simulink model "GFo_29bus"  (R2017b)
settings: Solver=ode1  StartTime=0.0  StopTime=4.5  FixedStep=Time_Step  RelTol=1e-3  EnableMultiTasking=on
PreLoadFcn:
  | Init_29bus;
InitFcn:
  | Init_29bus;
undefined symbols (not defined in the file): D1, D11, Delta, Time_Step, VSC01_Delta_P_Time_Step, VSC01_Delta_P_Value
libraries: powerlib x168, sps_avr x6, GFo_Lib x1
(part 1 of 5)
Description:
  | Copyright 2008-2017 The MathWorks, Inc.
settings Model: Creator=MathWorks  LastModifiedBy=Frederic_Colas
settings DataIOCC: SaveFormat=StructureWithTime  SignalLoggingSaveFormat=ModelDataLogs  SaveOutput=off  SignalLogging=off  DSMLogging=off  SaveTime=off
settings OptimizationCC: ExpressionDepthLimit=2147483647  LifeSpan=inf
settings DebuggingCC: UnderspecifiedInitializationDetection=Classic  MergeDetectMultiDrivingBlocksExec=none  SolverPrmCheckMsg=warning  FcnCallInpInsideContextMsg=warning  UnconnectedInputMsg=none  UnconnectedOutputMsg=none  UnconnectedLineMsg=none  StateNameClashWarn=warning  SFUnexpectedBacktrackingDiag=warning  SFNoUnconditionalDefaultTransitionDiag=warning  SFExecutionAtInitializationDiag=none
settings HardwareCC: ProdBitPerPointer=32  ProdBitPerSizeT=32  ProdBitPerPtrDiffT=32  ProdLargestAtomicFloat=None  ProdIntDivRoundTo=Undefined  ProdEndianess=Unspecified  ProdWordSize=32  ProdHWDeviceType=32-bit Generic
settings ModelReferenceCC: PropagateSignalLabelsOutOfModel=off
settings CodeAppCC: StateflowObjectComments=on
settings GRTTargetCC: TargetLangStandard=C89/C90 (ANSI)  GeneratePreprocessorConditionals=Disable all  CombineOutputUpdateFcns=off  GRTInterface=on
settings ConfigComp: CovMetricSettings=dw  CovHtmlReporting=on  CovSaveCumulativeToWorkspaceVar=on  CovSaveSingleToWorkspaceVar=on  CovExternalEMLEnable=off  CovSFcnEnable=off
settings SimscapeCC: SimscapeNormalizeSystem=off

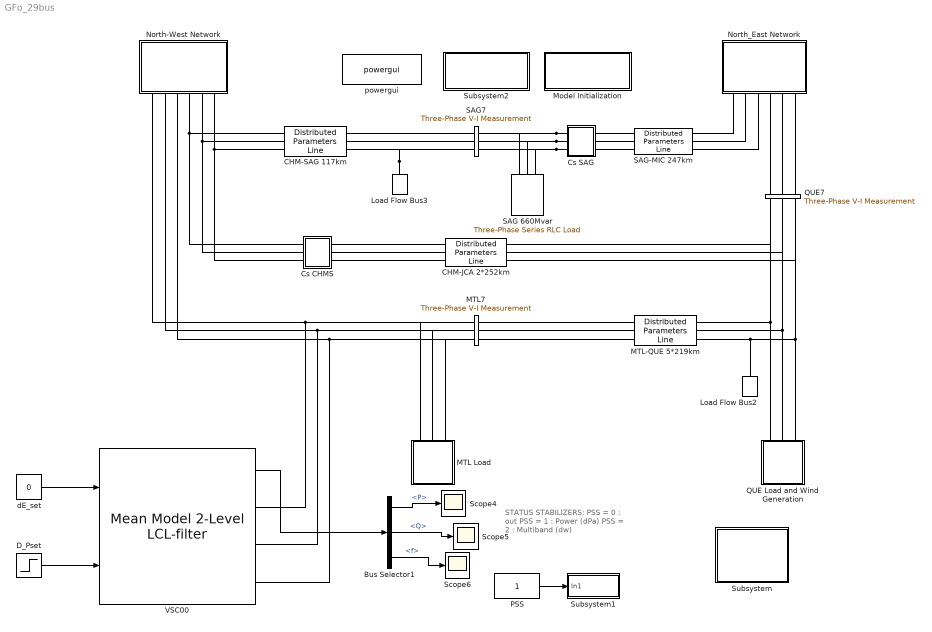
== system GFo_29bus ==
  note: STATUS STABILIZERS:
      | PSS = 0 :  out
      | PSS = 1 :  Power (dPa)
      | PSS = 2 :  Multiband (dw)
  Bus Selector1 : BusSelector  OutputSignals=control.P,control.Q,control.f
  CHM-JCA 2*252km : powerlib/Elements/Distributed Parameters Line  Phases=3  Frequency=60  Resistance="[0.01273  0.3864]/2"  Inductance="[0.9337e-3  4.1264e-3]/2"  Capacitance=[12.74e-9 7.751e-9]*2  Length=252  x1=[-0.00144 -1.85754414485872e-08 0 0;-0.0014 -1.70488676972424e-08 0 0;-0.00136 -1.55184171804064e-08 0 0;-0.00132 -1.39844379093287e-08 0 0;-0.00128 -1.2447278697667e-08 0 0;-0.00124 -1.09072890821703e-08 0 0;-0.0012 -9.36481924319672e-09 0 0;-0.00116 -7.82021992508601e-09 0 0;-0.00112 -6.27384235640306e-09 0 0;-0.00108 -4.72603817007156e-09 0 0;-0.00104 -3.17715932341582e-09 0 0;-0.001 -1.62755801812856e-09 0 0;-0.00096 -7.7586620183467e-11 0 0;-0.00092 1.47240242028999e-09 0 0;-0.00088 3.02205664915053e-09 172196.876340074 -778424.9668511;-0.00084 4.57102368839016e-09 183915.187892279 -775739.943274932;-0.0008 6.11895131626187e-09 195591.678716774 -772878.523125359;-0.00076 7.66548754737186e-09 207223.69368024 -769841.357064648;-0.00072 9.21028071271792e-09 218808.587762784 -766629.13571817;-0.00068 1.0752979539656e-08 230343.726659395 -763242.589517357;-0.00064 1.22932332317765e-08 241826.487378964 -759682.488533612;-0.0006 1.38306915486724e-08 253254.258840726 -755949.642303197;-0.00056 1.5365004885581e-08 264624.442467999 -752044.899643155;-0.00052 1.68958243528807e-08 275934.452779079 -747969.148458292;-0.00048 1.8422801855426e-08 287181.717975154 -743723.315539282;-0.00044 1.99455901717008e-08 298363.680525112 -739308.366351914;-0.0004 2.1463843032774e-08 309477.797747096 -734725.304817562;-0.00036 2.29772152010379e-08 320521.542386696 -729975.173084896;-0.00032 2.44853625487121e-08 331492.403191618 -725059.051292908;-0.00028 2.59879421360955e-08 342387.885482722 -719978.057325298;-0.00024 2.74846122895477e-08 353205.511721295 -714733.34655628;-0.0002 2.89750326791824e-08 363942.822072417 -709326.111587852;-0.00016 3.04588643962559e-08 374597.374964309 -703757.581978617;-0.00012 3.19357700302317e-08 385166.747643524 -698029.023964187;-8e-05 3.3405413745505e-08 395648.536725862 -692141.740169254;-4e-05 3.48674613577686e-08 406040.358742876 -686097.069311382]  x2=[-0.00144 -4.16824187889297e-09 0 0;-0.0014 -3.16521867758044e-09 0 0;-0.00136 -2.16147573283633e-09 0 0;-0.00132 -1.15724128715034e-09 0 0;-0.00128 -1.52743694775274e-10 0 0;-0.00124 8.51788630198777e-10 0 0;-0.0012 1.85612726578383e-09 0 0;-0.00116 2.86004383403521e-09 0 0;-0.00112 3.86331005298269e-09 0 0;-0.00108 4.8656977885399e-09 0 0;-0.00104 5.86697910637997e-09 0 0;-0.001 6.86692632376594e-09 0 0;-0.00096 7.86531206132372e-09 0 0;-0.00092 8.86190929474633e-09 0 0;-0.00088 9.85649140641716e-09 -50539.1882480982 -801013.244555649;-0.00084 1.08488322369409e-08 -38454.9386555758 -801684.296463899;-0.0008 1.18387061365704e-08 -26361.9447416245 -802173.052276564;-0.00076 1.2825888016517e-08 -14262.9563487746 -802479.400854788;-0.00072 1.38101534001344e-08 -2160.72468264951 -802603.272537544;-0.00068 1.47912784739624e-08 9941.99831363509 -802544.639157481;-0.00064 1.57690401386199e-08 22042.4605852394 -802303.514047325;-0.0006 1.67432160595363e-08 34137.9105913927 -801879.952036844;-0.00056 1.7713584717508e-08 46225.5979310702 -801274.049440389;-0.00052 1.86799254590705e-08 58302.7739684108 -800485.944034984;-0.00048 1.96420185466724e-08 70366.6924577328 -799515.815029002;-0.00044 2.05996452086424e-08 82414.6101680063 -798363.883021413;-0.0004 2.15525876889357e-08 94443.787506641 -797030.409951622;-0.00036 2.25006292966501e-08 106451.489142445 -795515.699039906;-0.00032 2.34435544552996e-08 118434.984627617 -793820.094718463;-0.00028 2.43811487518346e-08 130391.549018624 -791943.982553094;-0.00024 2.53131989853975e-08 142318.463495833 -789887.789155527;-0.0002 2.62394932158028e-08 154213.015981746 -787651.982086408;-0.00016 2.71598208117306e-08 166072.5017577 -785237.069748983;-0.00012 2.80739724986222e-08 177894.224078904 -782643.601273494;-8e-05 2.89817404062672e-08 189675.494787646 -779872.166392307;-4e-05 2.98829181160717e-08 201413.634924565 -776923.395305812]  x3=[-0.00144 6.24964800002417e-11 0 0;-0.0014 6.65040601264245e-11 0 0;-0.00136 7.0496517802841e-11 0 0;-0.00132 7.44729451790454e-11 0 0;-0.00128 7.84324380497433e-11 0 0;-0.00124 8.23740960604013e-11 0 0;-0.0012 8.62970229119791e-11 0 0;-0.00116 9.02003265647405e-11 0 0;-0.00112 9.40831194410956e-11 0 0;-0.00108 9.7944518627428e-11 0 0;-0.00104 1.01783646074862e-10 0 0;-0.001 1.05599628798924e-10 0 0;-0.00096 1.09391599078049e-10 0 0;-0.00092 1.13158694650896e-10 0 0;-0.00088 1.16900058912419e-10 -378.521018352371 -850.366045683333;-0.00084 1.20614841108649e-10 -365.655684342529 -855.977425052353;-0.0008 1.24302196530148e-10 -352.707203383348 -861.394162536551;-0.00076 1.27961286704093e-10 -339.678519847734 -866.615026416536;-0.00072 1.31591279584933e-10 -326.57259634597 -871.638829512882;-0.00068 1.3519134974359e-10 -313.392413052039 -876.464429456091;-0.00064 1.38760678555156e-10 -300.140967025961 -881.090728946349;-0.0006 1.42298454385039e-10 -286.821271532287 -885.516676003047;-0.00056 1.45803872773525e-10 -273.436355354908 -889.741264203993;-0.00052 1.49276136618702e-10 -259.989262108336 -893.763532914261;-0.00048 1.52714456357713e-10 -246.483049545612 -897.582567504632;-0.00044 1.56118050146303e-10 -232.920788863001 -901.197499559575;-0.0004 1.59486144036594e-10 -219.305564001625 -904.607507074715;-0.00036 1.6281797215308e-10 -205.640470946207 -907.811814643748;-0.00032 1.66112776866782e-10 -191.928617021063 -910.809693634768;-0.00028 1.6936980896752e-10 -178.17312018353 -913.600462355943;-0.00024 1.72588327834281e-10 -164.377108314967 -916.183486210533;-0.0002 1.75767601603632e-10 -150.543718509501 -918.558177841189;-0.00016 1.78906907336133e-10 -136.67609636068 -920.723997263512;-0.00012 1.82005531180733e-10 -122.777395246191 -922.680451988843;-8e-05 1.85062768537091e-10 -108.85077561081 -924.427097136249;-4e-05 1.88077924215798e-10 -94.8994042477446 -925.963535533686]  x4=[-0.00144 -2.38829442616442e-10 0 0;-0.0014 -2.36838630214904e-10 0 0;-0.00136 -2.34793962751264e-10 0 0;-0.00132 -2.32695905165271e-10 0 0;-0.00128 -2.30544934537127e-10 0 0;-0.00124 -2.28341539979005e-10 0 0;-0.0012 -2.26086222523825e-10 0 0;-0.00116 -2.23779495011327e-10 0 0;-0.00112 -2.21421881971456e-10 0 0;-0.00108 -2.19013919505086e-10 0 0;-0.00104 -2.16556155162116e-10 0 0;-0.001 -2.14049147816963e-10 0 0;-0.00096 -2.11493467541477e-10 0 0;-0.00092 -2.08889695475315e-10 0 0;-0.00088 -2.06238423693789e-10 -648.242255193202 -10861.6585886729;-0.00084 -2.0354025507324e-10 -484.384788092552 -10870.1989782703;-0.0008 -2.00795803153944e-10 -320.417176068246 -10876.2675783607;-0.00076 -1.980056920006e-10 -156.376703941262 -10879.8630089967;-0.00072 -1.95170556060423e-10 7.69932689966229 -10880.9844526083;-0.00068 -1.92291040018877e-10 171.773606980046 -10879.6316541891;-0.00064 -1.89367798653078e-10 335.808827223516 -10875.8049213537;-0.0006 -1.86401496682904e-10 499.767687435566 -10869.5051242681;-0.00056 -1.83392808619843e-10 663.612904785307 -10860.7336954518;-0.00052 -1.80342418613613e-10 827.307222283253 -10849.4926294522;-0.00048 -1.77251020296597e-10 990.813417253246 -10835.7844823907;-0.00044 -1.74119316626114e-10 1154.09430979657 -10819.6123713818;-0.0004 -1.70948019724571e-10 1317.11277124632 -10800.9799738239;-0.00036 -1.67737850717535e-10 1479.8317326102 -10779.8915265637;-0.00032 -1.64489539569756e-10 1642.2141929996 -10756.3518249321;-0.00028 -1.61203824919176e-10 1804.22322804337 -10730.3662216544;-0.00024 -1.57881453908972e-10 1965.82199828404 -10701.9406256326;-0.0002 -1.54523182017661e-10 2126.97375755482 -10671.0815006022;-0.00016 -1.5112977288731e-10 2287.64186133538 -10637.795863662;-0.00012 -1.47701998149892e-10 2447.78977508446 -10602.0912836789;-8e-05 -1.44240637251823e-10 2607.38108254751 -10563.9758795664;-4e-05 -1.40746477276721e-10 2766.3794940375 -10523.4583184387]  x5=0.00142516474882927  V1=ones(3,3)  V2=ones(3,3)  I1=ones(3,3)  I2=ones(3,3)  nHarmo=1  Measurements=None
      settings: AttributesFormatString=\n  SourceProductName=Simscape Power Systems
  CHM-SAG 117km : powerlib/Elements/Distributed Parameters Line  Phases=3  Frequency=60  Resistance="[0.01273  0.3864]"  Inductance="[0.9337e-3  4.1264e-3]"  Capacitance=[12.74e-9 7.751e-9]  Length=117  x1=[-0.00068 1.03484332071882e-08 0 0;-0.00064 1.18635422964804e-08 0 0;-0.0006 1.33759537185611e-08 0 0;-0.00056 1.48853235641156e-08 0 0;-0.00052 1.63913086154571e-08 0 0;-0.00048 1.78935664245721e-08 0 0;-0.00044 1.93917553909897e-08 223467.945952777 -779436.69611525;-0.0004 2.08855348394588e-08 235195.677690823 -775978.427940146;-0.00036 2.23745650974146e-08 246869.927960004 -772343.708962281;-0.00032 2.38585075722172e-08 258488.042136482 -768533.365685406;-0.00028 2.53370248281449e-08 270047.378361284 -764548.264548724;-0.00024 2.68097806631239e-08 281545.308141037 -760389.311729867;-0.0002 2.82764401851778e-08 292979.216945661 -756057.452938841;-0.00016 2.97366698885793e-08 304346.504802897 -751553.673202978;-0.00012 3.11901377296862e-08 315644.586889514 -746878.996642952;-8e-05 3.26365132024456e-08 326870.894119075 -742034.486239899;-4e-05 3.40754674135481e-08 338022.873726127 -737021.243593708]  x2=[-0.00068 7.57652475797684e-09 0 0;-0.00064 8.6127901811104e-09 0 0;-0.0006 9.64709713003032e-09 0 0;-0.00056 1.06792104122559e-08 0 0;-0.00052 1.17088953341273e-08 0 0;-0.00048 1.2735917754173e-08 0 0;-0.00044 1.37600441363512e-08 265658.843850609 -751135.268348524;-0.0004 1.47810416031544e-08 276955.015824463 -747044.008737732;-0.00036 1.57986779885633e-08 288188.210616077 -742782.877761587;-0.00032 1.68127218908396e-08 299355.873893826 -738352.844364525;-0.00028 1.78229427251446e-08 310455.466227387 -733754.915897938;-0.00024 1.88291107759725e-08 321484.463665181 -728990.137891109;-0.0002 1.98309972493853e-08 332440.358308303 -724059.593813467;-0.00016 2.08283743250387e-08 343320.658880788 -718964.404828216;-0.00012 2.1821015207987e-08 354122.891296115 -713705.729537391;-8e-05 2.28086941802533e-08 364844.599219787 -708284.763718406;-4e-05 2.37911866521568e-08 375483.344627883 -702702.740052139]  x3=[-0.00068 1.54291039105485e-10 0 0;-0.00064 1.55495560223311e-10 0 0;-0.0006 1.56664722991678e-10 0 0;-0.00056 1.57798261553056e-10 0 0;-0.00052 1.58895918150551e-10 0 0;-0.00048 1.59957443186519e-10 0 0;-0.00044 1.6098259527932e-10 1327.17874386151 -3929.54387650929;-0.0004 1.6197114131821e-10 1386.28134396302 -3909.08471567241;-0.00036 1.62922856516344e-10 1445.0687156417 -3887.73666268169;-0.00032 1.63837524461892e-10 1503.52749115618 -3865.50457190029;-0.00028 1.64714937167253e-10 1561.64437748503 -3842.39349871393;-0.00024 1.65554895116343e-10 1619.4061593495 -3818.40869838136;-0.0002 1.66357207309968e-10 1676.79970221849 -3793.55562483933;-0.00016 1.67121691309254e-10 1733.81195529531 -3767.83992946244;-0.00012 1.67848173277132e-10 1790.42995448525 -3741.26745977806;-8e-05 1.68536488017869e-10 1846.64082534354 -3713.84425813664;-4e-05 1.69186479014627e-10 1902.43178600291 -3685.57656033774]  x4=[-0.00068 -1.5758176037485e-10 0 0;-0.00064 -1.55417777405434e-10 0 0;-0.0006 -1.53218453773701e-10 0 0;-0.00056 -1.50984289586881e-10 0 0;-0.00052 -1.48715792874641e-10 0 0;-0.00048 -1.46413479473572e-10 0 0;-0.00044 -1.44077872909887e-10 42.4498796181136 -1838.17704499413;-0.0004 -1.41709504280376e-10 70.1631282495175 -1837.32799490434;-0.00036 -1.39308912131643e-10 97.8604223906187 -1836.06115227294;-0.00032 -1.3687664233764e-10 125.535463915581 -1834.37680516904;-0.00028 -1.34413247975544e-10 153.18195975862 -1832.27533659864;-0.00024 -1.31919289199988e-10 180.793623344995 -1829.75722441756;-0.0002 -1.29395333115692e-10 208.364176020519 -1826.8230412228;-0.00016 -1.26841953648503e-10 235.887348479272 -1823.47345422233;-0.00012 -1.24259731414893e-10 263.356882189187 -1819.70922508332;-8e-05 -1.21649253589929e-10 290.766530815185 -1815.53120975904;-4e-05 -1.19011113773758e-10 318.11006163954 -1810.94035829413]  x5=0.000661683633385019  V1=ones(3,3)  V2=ones(3,3)  I1=ones(3,3)  I2=ones(3,3)  nHarmo=1  Measurements=None
      settings: AttributesFormatString=\n  SourceProductName=Simscape Power Systems
  Cs CHMS : Subsystem  mask{Xc=33/2}
      mask prompts: Xc "Condensator Reactance at  60Hz  (ohm):"
      mask help: Series Compensation
      mask init:
      | Cs=1/Xc/(2*pi*60);
      mask Display: disp('Cs')
  Cs SAG : Subsystem  mask{Xc=22}
      mask prompts: Xc "Condensator Reactance at  60Hz  (ohm):"
      mask help: Series Compensation
      mask init:
      | Cs=1/Xc/(2*pi*60);
      mask Display: disp('Cs')
  D_Pset : Step  Time=VSC01_Delta_P_Time_Step  After=VSC01_Delta_P_Value  SampleTime=0
  Load Flow Bus2 : powerlib/Measurements/Load Flow Bus  LConnTagsString=a  Phases=single  Connectors=on one side  ID=QUE7  Vbase=735e3  Vref=1  Vangle=0  VLF=1.092  VLFb=1  VLFc=1  angleLF=-14.6  angleLFb=0  angleLFc=0
      settings: AttributesFormatString=%<ID>\n%<Vbase>V\n%<VLF>pu\n%<angleLF>deg.  SourceProductName=Simscape Power Systems
  Load Flow Bus3 : powerlib/Measurements/Load Flow Bus  LConnTagsString=a  Phases=single  Connectors=on one side  ID=SAG7  Vbase=735e3  Vref=1  Vangle=0  VLF=1.084  VLFb=1  VLFc=1  angleLF=-1.02  angleLFb=0  angleLFc=0
      settings: AttributesFormatString=%<ID>\n%<Vbase>V\n%<VLF>pu\n%<angleLF>deg.  SourceProductName=Simscape Power Systems
  MTL Load : Subsystem
  MTL-QUE 5*219km : powerlib/Elements/Distributed Parameters Line  Phases=3  Frequency=60  Resistance="[0.01273  0.3864]/5"  Inductance="[0.9337e-3  4.1264e-3]/5"  Capacitance=[12.74e-9 7.751e-9]*5  Length=219  x1=[-0.00124 -5.4468796144153e-08 -263340.269226421 -757862.009549339;-0.0012 -4.83459032566071e-08 -251882.489501348 -761746.813211586;-0.00116 -4.2212016927578e-08 -240367.433870303 -765458.402217534;-0.00112 -3.60685319499204e-08 -228797.720757637 -768995.932583849;-0.00108 -2.99168452991393e-08 -217175.981016339 -772358.599906634;-0.00104 -2.3758355815729e-08 -205504.857329803 -775545.639544336;-0.001 -1.75944638870895e-08 -193787.003610908 -778556.326791627;-0.00096 -1.14265711290903e-08 -182025.084398541 -781389.97704419;-0.00092 -5.25608006735493e-09 -170221.774251699 -784045.945954392;-0.00088 9.15606181661316e-10 -158379.757141321 -786523.629577809;-0.00084 7.08708422972765e-09 -146501.725839979 -788822.464510551;-0.0008 1.32569507359566e-08 -134590.381309558 -790941.928017378;-0.00076 1.94238027259112e-08 -122648.432087085 -792881.538150567;-0.00072 2.55862379106297e-08 -110678.593668831 -794640.8538595;-0.00068 3.17428550054937e-08 -98683.5878928278 -796219.475090956;-0.00064 3.78922540488681e-08 -86666.1423199488 -797617.04288008;-0.0006 4.40330367204407e-08 -74628.9896136833 -798833.23943201;-0.00056 5.01638066591878e-08 -62574.8669187526 -799867.788194138;-0.00052 5.62831697808949e-08 -50506.5152387072 -800720.453918996;-0.00048 6.23897345951591e-08 -38426.6788126462 -801391.042717752;-0.00044 6.84821125218026e-08 -26338.1044912007 -801879.402104296;-0.0004 7.45589182066232e-08 -14243.5411119241 -802185.421029915;-0.00036 8.06187698364124e-08 -2145.73887422974 -802309.029908544;-0.00032 8.66602894531674e-08 9952.55128598059 -802250.200632591;-0.00028 9.26821032674272e-08 22048.5783218556 -802008.946579325;-0.00024 9.86828419706605e-08 34139.5917011591 -801585.322607837;-0.0002 1.04661141046634e-07 46222.8420317171 -800979.425046565;-0.00016 1.10615641081693e-07 58295.5816866058 -800191.391671391;-0.00012 1.16544988073879e-07 70355.0654289387 -799221.401674307;-8e-05 1.22447833740818e-07 82398.5510361093 -798069.675622674;-4e-05 1.28322835826309e-07 94423.2999233492 -796736.475409064]  x2=[-0.00124 9.0375128968403e-10 -158451.694559255 -786809.273834629;-0.0012 1.9084795416908e-09 -146569.352833624 -789109.165478305;-0.00116 2.91277382190782e-09 -134653.682501119 -791229.620502738;-0.00112 3.91640576247643e-09 -122707.393082416 -793170.156734742;-0.00108 4.91914714614829e-09 -110733.201060711 -794930.332913113;-0.00104 5.92076995818004e-09 -98733.8292640061 -796509.748788967;-0.001 6.92104643818184e-09 -86712.0062459713 -797908.045216754;-0.00096 7.91974913190816e-09 -74670.4656654886 -799124.904235924;-0.00092 8.91665094297889e-09 -62611.9456650443 -800160.049143231;-0.00088 9.91152518451912e-09 -50539.1882480981 -801013.244555649;-0.00084 1.09041456307057e-08 -38454.9386555758 -801684.296463899;-0.0008 1.18942865682093e-08 -26361.9447416244 -802173.052276565;-0.00076 1.28817228475192e-08 -14262.9563487745 -802479.400854788;-0.00072 1.38662299341408e-08 -2160.72468264948 -802603.272537544;-0.00068 1.48475839596526e-08 9941.99831363515 -802544.639157482;-0.00064 1.58255617726122e-08 22042.4605852394 -802303.514047325;-0.0006 1.67999409892985e-08 34137.9105913927 -801879.952036844;-0.00056 1.77705000442803e-08 46225.5979310702 -801274.049440389;-0.00052 1.87370182407984e-08 58302.7739684108 -800485.944034984;-0.00048 1.96992758009496e-08 70366.6924577328 -799515.815029002;-0.00044 2.0657053915663e-08 82414.6101680063 -798363.883021413;-0.0004 2.16101347944549e-08 94443.787506641 -797030.409951622;-0.00036 2.25583017149523e-08 106451.489142445 -795515.699039906;-0.00032 2.35013390721743e-08 118434.984627617 -793820.094718463;-0.00028 2.44390324275582e-08 130391.549018624 -791943.982553094;-0.00024 2.53711685577213e-08 142318.463495833 -789887.789155527;-0.0002 2.6297535502946e-08 154213.015981746 -787651.982086408;-0.00016 2.72179226153777e-08 166072.5017577 -785237.069748984;-0.00012 2.81321206069239e-08 177894.224078904 -782643.601273495;-8e-05 2.90399215968453e-08 189675.494787646 -779872.166392307;-4e-05 2.99411191590251e-08 201413.634924565 -776923.395305813]  x3=[-0.00124 3.81189466927696e-09 -8469.52016261608 -20114.2598393833;-0.0012 3.84351344492956e-09 -8165.25294654191 -20239.6869599555;-0.00116 3.87425823876983e-09 -7859.12902236185 -20360.5117502527;-0.00112 3.90412205969678e-09 -7551.21800001634 -20476.7067357594;-0.00108 3.93309811693508e-09 -7241.58989581657 -20588.245494738;-0.00104 3.96117982157917e-09 -6930.31511652329 -20695.1026642366;-0.001 3.9883607880916e-09 -6617.46444333701 -20797.2539458563;-0.00096 4.01463483575498e-09 -6303.10901580289 -20894.6761112766;-0.00092 4.03999599007744e-09 -5987.32031563429 -20987.3470075372;-0.00088 4.0644384841512e-09 -5670.17015045835 -21075.2455620755;-0.00084 4.08795675996389e-09 -5351.73063748767 -21158.3517875181;-0.0008 4.1105454696624e-09 -5032.07418712138 -21236.6467862261;-0.00076 4.13219947676895e-09 -4711.2734864797 -21310.112754592;-0.00072 4.15291385734904e-09 -4389.40148287549 -21378.732987088;-0.00068 4.17268390113118e-09 -4066.53136722666 -21442.4918800651;-0.00064 4.1915051125779e-09 -3742.73655741319 -21501.3749353009;-0.0006 4.20937321190802e-09 -3418.09068158255 -21555.3687632963;-0.00056 4.22628413606983e-09 -3092.66756140728 -21604.4610863206;-0.00052 4.24223403966503e-09 -2766.54119529857 -21648.6407412027;-0.00048 4.25721929582308e-09 -2439.78574157969 -21687.8976818703;-0.00044 4.27123649702595e-09 -2112.47550162299 -21722.2229816334;-0.0004 4.28428245588297e-09 -1784.68490295443 -21751.608835215;-0.00036 4.2963542058556e-09 -1456.48848232941 -21776.0485605253;-0.00032 4.307449001932e-09 -1127.96086878373 -21795.5366001817;-0.00028 4.31756432125122e-09 -799.176766663608 -21810.0685227718;-0.00024 4.32669786367688e-09 -470.210938638553 -21819.6410238619;-0.0002 4.33484755232019e-09 -141.138188700978 -21824.2519267477;-0.00016 4.34201153401224e-09 187.966654843584 -21823.9001829498;-0.00012 4.34818817972536e-09 517.02875639179 -21818.5858724515;-8e-05 4.35337608494359e-09 845.973290059458 -21808.3102036813;-4e-05 4.35757406998203e-09 1174.72545669633 -21793.0755132376]  x4=[-0.00124 -4.87811680086981e-09 -3328.85135662787 -7082.90675391454;-0.0012 -4.86617754969349e-09 -3221.66969661535 -7132.29763529397;-0.00116 -4.85313177170651e-09 -3113.75545669631 -7180.06669369745;-0.00112 -4.83898243340626e-09 -3005.13317563831 -7226.20306685304;-0.00108 -4.82373275223026e-09 -2895.82755321133 -7270.69626374736;-0.00104 -4.80738619582451e-09 -2785.8634445713 -7313.5361670111;-0.001 -4.78994648125495e-09 -2675.26585460824 -7354.71303521972;-0.00096 -4.7714175741623e-09 -2564.05993226035 -7394.21750510848;-0.00092 -4.75180368786024e-09 -2452.27096479538 -7432.04059370159;-0.00088 -4.73110928237737e-09 -2339.9243720605 -7468.17370035488;-0.00084 -4.70933906344303e-09 -2227.04570070206 -7502.6086087115;-0.0008 -4.68649798141728e-09 -2113.6606183565 -7535.33748857023;-0.00076 -4.66259123016519e-09 -1999.79490781376 -7566.35289766605;-0.00072 -4.63762424587583e-09 -1885.47446115448 -7595.64778336239;-0.00068 -4.61160270582614e-09 -1770.72527386238 -7623.21548425487;-0.00064 -4.5845325270899e-09 -1655.57343891308 -7649.04973168604;-0.0006 -4.55641986519233e-09 -1540.04514084083 -7673.14465117082;-0.00056 -4.52727111271031e-09 -1424.16664978434 -7695.4947637323;-0.00052 -4.49709289781877e-09 -1307.96431551318 -7716.09498714764;-0.00048 -4.46589208278356e-09 -1191.46456143607 -7734.94063710366;-0.00044 -4.43367576240093e-09 -1074.69387859244 -7752.02742826209;-0.0004 -4.40045126238432e-09 -957.678819628593 -7767.35147523398;-0.00036 -4.36622613769852e-09 -840.445992759828 -7780.90929346318;-0.00032 -4.33100817084174e-09 -723.022055720008 -7792.69780001875;-0.00028 -4.29480537007593e-09 -605.433709699793 -7802.71431429596;-0.00024 -4.25762596760579e-09 -487.707693275031 -7810.95655862585;-0.0002 -4.21947841770682e-09 -369.87077632663 -7817.42265879312;-0.00016 -4.1803713948029e-09 -251.949753953322 -7822.11114446236;-0.00012 -4.14031379149379e-09 -133.971440378687 -7825.02094951237;-8e-05 -4.09931471653303e-09 -15.96266285383 -7826.15141227857;-4e-05 -4.05738349275672e-09 102.049744442903 -7825.50227570347]  x5=0.00123853603172068  V1=ones(3,3)  V2=ones(3,3)  I1=ones(3,3)  I2=ones(3,3)  nHarmo=1  Measurements=None
      settings: AttributesFormatString=\n  SourceProductName=Simscape Power Systems
  MTL7 : powerlib/Measurements/Three-Phase V-I Measurement  VoltageMeasurement=phase-to-ground  SetLabelV=on  LabelV=Vabc_MTL7  Vpu=on  VpuLL=off  CurrentMeasurement=no  SetLabelI=off  LabelI=A1  Ipu=off  Pbase=100e6  Vbase=735e3  OutputType=Magnitude  PhasorSimulation=off  PSBequivalent=0
  Model Initialization : Subsystem  mask(Model Functions){InitFcnX=Init_29bus;, prel=on, posl=off, inif=on, strf=off}
      mask prompts: InitFcnX "Initialisation"; prel "Preload Function"; posl "PostLoad Function"; inif "InitFcn"; strf "StartFcn"
      mask init:
      | currentBlock = gcb;
      | root = bdroot(currentBlock);
      | 
      | if ~strcmp(get_param(root,'BlockDiagramType'),'library')
      |     if prel==1
      |         set_param(root, 'PreLoadFcn', InitFcnX);
      |     else
      |         set_param(root, 'PreLoadFcn', '');
      |     end
      |     if inif==1
      |         set_param(root, 'InitFcn', InitFcnX);
      |     else
      |         set_param(root, 'InitFcn', '');
      |     end
      |     if strf==1
      |         set_param(root, 'StartFcn', InitFcnX);
      |     else
      |         set_param(root, 'StartFcn', '');
      |     end
      |     if posl==1
      |         set_param(root, 'PostLoadFcn', InitFcnX);
      |     else
      |         set_param(root, 'PostLoadFcn', '');
      |     end
      | end
      | 
      | pos = get_param(currentBlock, 'Position');
      | width = pos(3) - pos(1); height = pos(4) - pos(2);
      | txt = [ upper(root) '\n' '- InitFcn. . . . . '  get_param(root, 'InitFcn') ];
      settings: CopyFcn=set_param(gcb,'LinkStatus','none')
      mask Display:
      | %text(5, height*0.5, txt, 'horizontalAlignment', 'left', 'verticalAlignment', 'middle') ;
      | color('blue'),disp('Initialization Function\nParameters')
  North-West Network : Subsystem
  North_East Network : Subsystem
  PSS : Constant
  QUE Load and Wind Generation : Subsystem
  QUE7 : powerlib/Measurements/Three-Phase V-I Measurement  VoltageMeasurement=no  SetLabelV=on  LabelV=Vabc_QUE7  Vpu=on  VpuLL=off  CurrentMeasurement=no  SetLabelI=off  LabelI=A1  Ipu=off  Pbase=100e6  Vbase=735e3  OutputType=Magnitude  PhasorSimulation=off  PSBequivalent=0
  SAG 660Mvar : powerlib/Elements/Three-Phase Series RLC Load  LConnTagsString=A|B|C  Configuration=Y (grounded)  NominalVoltage=735e3  Vabc=[1e3 1e3 1e3]  Vabcp=[1e3 1e3 1e3]  NominalFrequency=60  UnbalancedPower=off  ActivePower=2200000  InductivePower=660e6  CapacitivePower=0  Pabc=[10e3 9e3 11e3]  QLabc=[100 90 110]  QCabc=[100 90 110]  Pabcp=[10e3 9e3 11e3]  QLabcp=[100 90 110]  QCabcp=[100 90 110]  Measurements=None  LoadType=constant Z
  SAG-MIC 247km : powerlib/Elements/Distributed Parameters Line  Phases=3  Frequency=60  Resistance="[0.01273  0.3864]/1"  Inductance="[0.9337e-3  4.1264e-3]/1"  Capacitance=[12.74e-9 7.751e-9]*1  Length=247  x1=[-0.0014 -1.08735468814976e-08 -43484.2882453679 -787188.223839926;-0.00136 -9.81375428176395e-09 -31609.3049024198 -787754.475242769;-0.00132 -8.75173011893683e-09 -19727.1338761239 -788141.598071246;-0.00128 -7.68771588815238e-09 -7840.47706970408 -788349.504296966;-0.00124 -6.62195353707101e-09 4047.96259358793 -788378.146643845;-0.0012 -5.55468541086059e-09 15935.4817850944 -788227.518598861;-0.00116 -4.48615419708932e-09 27819.3773854646 -787897.654413532;-0.00112 -3.41660287054057e-09 39696.9470993214 -787388.62909613;-0.00108 -2.3462746379626e-09 51565.4900697397 -786700.558394621;-0.00104 -1.27541288276536e-09 63422.307492398 -785833.59877035;-0.001 -2.04261109677269e-10 75264.7032292633 -784787.947362459;-0.00096 8.66937110625693e-10 87089.9844216694 -783563.841943061;-0.00092 1.93793819690584e-09 98895.46210265 -782161.560863172;-0.00088 3.00849861275208e-09 110678.451808387 -780581.422989417;-0.00084 4.07837492195797e-09 122436.274188632 -778823.787631521;-0.0008 5.14732384387701e-09 134166.255615973 -776889.054460608;-0.00076 6.21510230874259e-09 145865.728793787 -774777.663418317;-0.00072 7.28146751293991e-09 157532.033362766 -772490.094616762;-0.00068 8.34617697421749e-09 169162.516505857 -770026.868229362;-0.00064 9.40898858682551e-09 180754.533551489 -767388.544372556;-0.0006 1.04696606765685e-08 192305.448574953 -764575.722978437;-0.00056 1.15279520557602e-08 203812.634997782 -761589.043658332;-0.00052 1.25836220780673e-08 215273.476185018 -758429.185557364;-0.00048 1.36364306932303e-08 226685.366040209 -755096.867200015;-0.00044 1.46861385016492e-08 238045.709598014 -751592.846326742;-0.0004 1.57325068088207e-08 249351.923614275 -747917.919721676;-0.00036 1.67752976796153e-08 260601.437153426 -744072.923031434;-0.00032 1.78142739923815e-08 271791.692173099 -740058.730575107;-0.00028 1.88491994928657e-08 282920.144105803 -735876.255145441;-0.00024 1.98798388479337e-08 293984.262437537 -731526.447801282;-0.0002 2.09059576990841e-08 304981.531283206 -727010.297651308;-0.00016 2.1927322715739e-08 315909.449958709 -722328.831629118;-0.00012 2.29437016483016e-08 326765.533549578 -717483.114259714;-8e-05 2.39548633809674e-08 337547.313476025 -712474.247417439;-4e-05 2.49605779842783e-08 348252.338054271 -707303.370075417]  x2=[-0.0014 -1.04301270405993e-09 59840.985994314 -786906.914710697;-0.00136 -6.98506067436651e-10 71699.9647213889 -785915.133906567;-0.00132 -3.53840596557298e-10 83542.6394948002 -784744.642778429;-0.00128 -9.09466537767774e-12 95366.3173924316 -783395.707485873;-0.00124 3.35653333850417e-10 107168.309811892 -781868.634765151;-0.0012 6.80325008404946e-10 118945.933081881 -780163.771859432;-0.00116 1.02484198291944e-09 130696.509072434 -778281.506439838;-0.00112 1.36912591720487e-09 142417.365803902 -776222.266517293;-0.00108 1.71309852406357e-09 154105.838054541 -773986.520345198;-0.00104 2.05668158709104e-09 165759.267966559 -771574.776312952;-0.001 2.39979697846166e-09 177375.005650489 -768987.58283035;-0.00096 2.74236667669435e-09 188950.40978775 -766225.528202878;-0.00092 3.08431278439393e-09 200482.848231265 -763289.240497941;-0.00088 3.42555754596431e-09 211969.698603982 -760179.387402041;-0.00084 3.76602336528949e-09 223408.348895185 -756896.676068953;-0.0008 4.10563282337821e-09 234796.198054442 -753441.852958926;-0.00076 4.44430869596836e-09 246130.656583056 -749815.703668943;-0.00072 4.78197397108713e-09 257409.147122905 -746019.05275408;-0.00068 5.11855186656286e-09 268629.105042499 -742052.763540015;-0.00064 5.45396584748465e-09 279787.979020166 -737917.737926711;-0.0006 5.78813964360572e-09 290883.231624192 -733614.916183335;-0.00056 6.12099726668663e-09 301912.339889817 -729145.276734444;-0.00052 6.45246302777432e-09 312872.795892932 -724509.835937505;-0.00048 6.78246155441317e-09 323762.107320361 -719709.64785178;-0.00044 7.110917807784e-09 334577.798036591 -714745.803998646;-0.0004 7.43775709976728e-09 345317.408646824 -709619.433113387;-0.00036 7.76290510992657e-09 355978.49705622 -704331.700888536;-0.00032 8.08628790240829e-09 366558.639025214 -698883.809708801;-0.00028 8.40783194275419e-09 377055.428720761 -693276.998377655;-0.00024 8.72746411462236e-09 387466.479263404 -687512.541835644;-0.0002 9.04511173641331e-09 397789.423270032 -681591.750870476;-0.00016 9.36070257779712e-09 408021.913392197 -675515.971818956;-0.00012 9.674164876138e-09 418161.622849888 -669286.586260847;-8e-05 9.98542735281249e-09 428206.245960616 -662905.010704703;-4e-05 1.02944192294176e-08 438153.498663705 -656372.696265775]  x3=[-0.0014 8.14598994752012e-11 -581.71165728291 -4056.93337045252;-0.00136 8.26501374952971e-11 -520.470981275651 -4065.24415192315;-0.00132 8.3821581586871e-11 -459.1119546556 -4072.63053193081;-0.00128 8.49739653736386e-11 -397.648529936272 -4079.09083087638;-0.00124 8.61070268134644e-11 -336.094683370413 -4084.62357974358;-0.0012 8.72205082579483e-11 -274.464411771912 -4089.22752043305;-0.00116 8.83141565110119e-11 -212.771729333055 -4092.90160604837;-0.00112 8.93877228864738e-11 -151.030664437812 -4095.64500113415;-0.00108 9.04409632645982e-11 -89.2552564719097 -4097.45708186601;-0.00104 9.14736381476058e-11 -27.4595526303898 -4098.33743619242;-0.001 9.24855127141338e-11 34.3423952765968 -4098.2858639284;-0.00096 9.34763568726316e-11 96.1365340190545 -4097.30237680103;-0.00092 9.44459453136824e-11 157.908812142722 -4095.38719844681;-0.00088 9.5394057561236e-11 219.645183164256 -4092.54076436077;-0.00084 9.63204780227435e-11 281.331608765277 -4088.76372179749;-0.0008 9.7224996038181e-11 342.954061984566 -4084.05692962387;-0.00076 9.81074059279522e-11 404.49853040767 -4078.42145812386;-0.00072 9.89675070396575e-11 465.951019353205 -4071.85858875508;-0.00068 9.98051037937215e-11 527.29755505513 -4064.36981385743;-0.00064 1.00620005727865e-10 588.524187840257 -4055.95683631374;-0.0006 1.01412027540417e-10 649.616995300284 -4046.62156916256;-0.00056 1.02180989132445e-10 710.562085457639 -4036.36613516313;-0.00052 1.02926715648716e-10 771.345599924387 -4025.1928663127;-0.00048 1.03649037517451e-10 831.953717053513 -4013.10430331625;-0.00044 1.04347790488886e-10 892.372655081845 -4000.10319500877;-0.0004 1.05022815672621e-10 952.588675263905 -3986.19249773016;-0.00036 1.05673959573749e-10 1012.58808499598 -3971.37537465304;-0.00032 1.06301074127765e-10 1072.35724092972 -3955.65519506339;-0.00028 1.06904016734224e-10 1131.88255207449 -3939.03553359451;-0.00024 1.0748265028918e-10 1191.15048288786 -3921.52016941408;-0.0002 1.08036843216351e-10 1250.14755635346 -3903.11308536488;-0.00016 1.08566469497044e-10 1308.86035704556 -3883.81846705908;-0.00012 1.09071408698811e-10 1367.27553417959 -3863.6407019265;-8e-05 1.09551546002832e-10 1425.37980464804 -3842.58437821691;-4e-05 1.10006772230024e-10 1483.15995604086 -3820.65428395676]  x4=[-0.0014 -1.28900997554246e-10 -294.730337180683 -1716.44188763853;-0.00136 -1.28413364013615e-10 -268.814439627778 -1720.69097664942;-0.00132 -1.27896530381396e-10 -242.837415989459 -1724.54879537083;-0.00128 -1.27350614181102e-10 -216.805173216884 -1728.01446656804;-0.00124 -1.26775739549367e-10 -190.723630817569 -1731.08720217732;-0.0012 -1.26172037207727e-10 -164.598719509335 -1733.76630348508;-0.00116 -1.25539644432887e-10 -138.436379871725 -1736.05116128679;-0.00112 -1.2487870502551e-10 -112.242560995156 -1737.9412560255;-0.00108 -1.24189369277519e-10 -86.0232191281554 -1739.43615790995;-0.00104 -1.23471793937918e-10 -59.7843163229576 -1740.53552701235;-0.001 -1.2272614217715e-10 -33.5318190797861 -1741.23911334565;-0.00096 -1.21952583549997e-10 -7.27169699012172 -1741.54675692038;-0.00092 -1.21151293957018e-10 18.9900786207295 -1741.45838778105;-0.00088 -1.20322455604558e-10 45.2475360514661 -1740.97402602203;-0.00084 -1.19466256963311e-10 71.4947045827026 -1740.09378178301;-0.0008 -1.18582892725462e-10 97.725615834661 -1738.81785522395;-0.00076 -1.17672563760424e-10 123.934305124329 -1737.14653647954;-0.00072 -1.16735477069151e-10 150.114812821775 -1735.08020559324;-0.00068 -1.15771845737077e-10 176.26118570532 -1732.61933243089;-0.00064 -1.14781888885656e-10 202.367478315248 -1729.76447657381;-0.0006 -1.13765831622539e-10 228.42775430575 -1726.51628719162;-0.00056 -1.12723904990386e-10 254.436087794799 -1722.87550289456;-0.00052 -1.11656345914328e-10 280.386564711648 -1718.84295156559;-0.00048 -1.10563397148092e-10 306.273284141632 -1714.4195501721;-0.00044 -1.09445307218802e-10 332.09035966799 -1709.60630455743;-0.0004 -1.08302330370468e-10 357.831920710385 -1704.40430921211;-0.00036 -1.07134726506166e-10 383.492113859822 -1698.81474702504;-0.00032 -1.05942761128948e-10 409.065104209662 -1692.83888901445;-0.00028 -1.0472670528146e-10 434.545076682432 -1686.47809403892;-0.00024 -1.03486835484316e-10 459.926237352121 -1679.73380848838;-0.0002 -1.02223433673216e-10 485.202814761672 -1672.60756595519;-0.00016 -1.00936787134835e-10 510.369061235357 -1665.10098688545;-0.00012 -9.96271884415017e-11 535.419254185752 -1657.21577821052;-8e-05 -9.82949353846651e-11 560.347697415004 -1648.95373295884;-4e-05 -9.69403309071814e-11 585.148722410097 -1640.31672984826]  x5=0.00139688767047948  V1=ones(3,3)  V2=ones(3,3)  I1=ones(3,3)  I2=ones(3,3)  nHarmo=1  Measurements=None
      settings: AttributesFormatString=\n  SourceProductName=Simscape Power Systems
  SAG7 : powerlib/Measurements/Three-Phase V-I Measurement  VoltageMeasurement=no  SetLabelV=on  LabelV=Vabc_SAG7  Vpu=on  VpuLL=off  CurrentMeasurement=no  SetLabelI=off  LabelI=Iabc_SAG7  Ipu=off  Pbase=100e6  Vbase=735e3  OutputType=Magnitude  PhasorSimulation=off  PSBequivalent=0
  Scope4 : Scope
  Scope5 : Scope
  Scope6 : Scope
  Subsystem : Subsystem
      mask Display: disp('Display\nWaveforms')
  Subsystem1 : Subsystem
      mask Display: disp('PSS_select')
  Subsystem2 : Subsystem
      settings: OpenFcn=LoadFlow_VSC
      mask Display: color('blue'),disp('Update Loadflow')
  VSC00 : GFo_Lib/Mean Model 2-Level LCL-filter  fn=fb  Sn=VSC01_Sn  Pn=VSC01_Pn  Udcn=VSC01_Udc_n  Un1=VSC01_Un1  Un2=VSC01_Un2  Rt_pu=VSC01_Rt_pu  Lt_pu=VSC01_Lt_pu  Rm_pu=500  Lm_pu=500  Lf_pu=VSC01_Lf_pu  Rf_pu=VSC01_Rf_pu  Cf_pu=VSC01_Cf_pu  Tr_PLL=VSC01_Tr_PLL  Val_Freq_Support=on  Val_gamma=on  R_percent=VSC01_R  Rv=VSC01_Rv  W_TVR=VSC01_W_LF  I_thresh_pu=1  DX_DR=5  Kp_Rvi_pu=0.676  gainpopup=3  wc1=VSC01_wc1  mp1=VSC01_mp1  wc2=VSC01_wc2  mp2=VSC01_mp2  wc3=VSC01_wc3  mp3=VSC01_mp3  T1=VSC01_T1  T2=VSC01_T2  LFpopup=PQ  P0=0.9  Q0=-0.3  V0=1.0915  Theta0=-22.3793  innercontrol=1  Kp_i=0.73  Ki_i=1.19  Kp_v=0.52  Ki_v=1.16  Kffv=1  Kffi=1  I_max=1.25
      settings: SourceProductName=VSC4SPS
  dE_set : Constant  Value=0
  powergui : powerlib/powergui  Priority=1  SimulationMode=Discrete  SampleTime=Time_Step  frequency=60  Iterations=50  frequencyindice=60  Pbase=1e+008  ErrMax=0.0001  UnitsV=kV  UnitsW=MW  buscounter=0  FunctionMessages=off  echomessages=off  EnableUseOfTLC=off  CurrentSourceSwitches=off  DisableSnubberDevices=off  DisableRonSwitches=off  DisableVfSwitches=off  DisplayEquations=off  SolverType=Tustin/Backward Euler (TBE)  Interpol=off  ExternalGateDelay=off  methode=off  Ts=100  x0status=blocks  SPID=off  SwTol=0  HookPort=off  RestoreLinks=warning  ResistiveCurrentMeasurement=off  Frange=[0:2:500]  Ylog=off  Xlog=on  ShowGrid=off  save=off  variable=ZData  structure=0  ZoomFFT=off  StartTime=0.0  cycles=1  DisplayStyle=1  fundamental=60  FreqAxis=off  MaxFrequency=1000  frequencyindicesteady=1  RmsSteady=1  display=off
  wires:
  PSS/1 -> Subsystem1/1(In1)
  D_Pset/1 -> VSC00/2
  dE_set/1 -> VSC00/1
  Bus Selector1/3 -> Scope6/1  "<f>"
  Bus Selector1/2 -> Scope5/1  "<Q>"
  VSC00/1 -> Bus Selector1/1
  Bus Selector1/1 -> Scope4/1  "<P>"
  connections:
  QUE Load and Wind Generation/LConn3 -- MTL-QUE 5*219km/RConn3 -- Load Flow Bus2/LConn1 -- CHM-JCA 2*252km/RConn3 -- QUE7/LConn3
  MTL7/RConn1 -- MTL-QUE 5*219km/LConn1
  MTL7/RConn2 -- MTL-QUE 5*219km/LConn2
  MTL7/RConn3 -- MTL-QUE 5*219km/LConn3
  QUE Load and Wind Generation/LConn2 -- MTL-QUE 5*219km/RConn2 -- CHM-JCA 2*252km/RConn2 -- QUE7/LConn2
  QUE Load and Wind Generation/LConn1 -- MTL-QUE 5*219km/RConn1 -- CHM-JCA 2*252km/RConn1 -- QUE7/LConn1
  Cs SAG/LConn1 -- SAG7/RConn1 -- SAG 660Mvar/LConn1
  Cs SAG/LConn2 -- SAG7/RConn2 -- SAG 660Mvar/LConn2
  Cs SAG/LConn3 -- SAG7/RConn3 -- SAG 660Mvar/LConn3
  Load Flow Bus3/LConn1 -- CHM-SAG 117km/RConn3 -- SAG7/LConn3
  Cs CHMS/LConn1 -- CHM-SAG 117km/LConn1 -- North-West Network/RConn4
  Cs CHMS/LConn2 -- CHM-SAG 117km/LConn2 -- North-West Network/RConn5
  Cs CHMS/LConn3 -- CHM-SAG 117km/LConn3 -- North-West Network/RConn6
  Cs SAG/RConn1 -- SAG-MIC 247km/LConn1
  Cs SAG/RConn3 -- SAG-MIC 247km/LConn3
  Cs CHMS/RConn3 -- CHM-JCA 2*252km/LConn3
  Cs CHMS/RConn2 -- CHM-JCA 2*252km/LConn2
  Cs CHMS/RConn1 -- CHM-JCA 2*252km/LConn1
  Cs SAG/RConn2 -- SAG-MIC 247km/LConn2
  SAG7/LConn2 -- CHM-SAG 117km/RConn2
  SAG7/LConn1 -- CHM-SAG 117km/RConn1
  SAG-MIC 247km/RConn1 -- North_East Network/LConn1
  SAG-MIC 247km/RConn2 -- North_East Network/LConn2
  SAG-MIC 247km/RConn3 -- North_East Network/LConn3
  QUE7/RConn1 -- North_East Network/LConn4
  QUE7/RConn2 -- North_East Network/LConn5
  QUE7/RConn3 -- North_East Network/LConn6
  MTL7/LConn1 -- MTL Load/LConn1 -- VSC00/RConn1 -- North-West Network/RConn1
  MTL7/LConn2 -- MTL Load/LConn2 -- VSC00/RConn2 -- North-West Network/RConn2
  MTL7/LConn3 -- MTL Load/LConn3 -- VSC00/RConn3 -- North-West Network/RConn3

== system GFo_29bus/Cs CHMS ==
  note: B
  Ca : powerlib/Elements/Series RLC Branch  LConnTagsString=__new0  RConnTagsString=__new0  BranchType=C  Resistance=1.0  Inductance=1.0  SetiL0=off  InitialCurrent=0  Capacitance=Cs  Setx0=off  InitialVoltage=0  Measurements=None
  Cb : powerlib/Elements/Series RLC Branch  LConnTagsString=__new0  RConnTagsString=__new0  BranchType=C  Resistance=1.0  Inductance=1.0  SetiL0=off  InitialCurrent=0  Capacitance=Cs  Setx0=off  InitialVoltage=0  Measurements=None
  Cc : powerlib/Elements/Series RLC Branch  LConnTagsString=__new0  RConnTagsString=__new0  BranchType=C  Resistance=1.0  Inductance=1.0  SetiL0=off  InitialCurrent=0  Capacitance=Cs  Setx0=off  InitialVoltage=0  Measurements=None
  A : PMIOPort  Port=1  Side=Left
  B : PMIOPort  Port=2  Side=Left
  C : PMIOPort  Port=3  Side=Left
  "A " : PMIOPort  Port=4  Side=Right
  "B " : PMIOPort  Port=5  Side=Right
  "C " : PMIOPort  Port=6  Side=Right
  connections:
  Cc/RConn1 -- "C "/RConn1
  C/RConn1 -- Cc/LConn1
  Cb/RConn1 -- "B "/RConn1
  B/RConn1 -- Cb/LConn1
  Ca/RConn1 -- "A "/RConn1
  A/RConn1 -- Ca/LConn1

== system GFo_29bus/Cs SAG ==
  note: B
  Ca : powerlib/Elements/Series RLC Branch  LConnTagsString=__new0  RConnTagsString=__new0  BranchType=C  Resistance=1.0  Inductance=1.0  SetiL0=off  InitialCurrent=0  Capacitance=Cs  Setx0=off  InitialVoltage=0  Measurements=None
  Cb : powerlib/Elements/Series RLC Branch  LConnTagsString=__new0  RConnTagsString=__new0  BranchType=C  Resistance=1.0  Inductance=1.0  SetiL0=off  InitialCurrent=0  Capacitance=Cs  Setx0=off  InitialVoltage=0  Measurements=None
  Cc : powerlib/Elements/Series RLC Branch  LConnTagsString=__new0  RConnTagsString=__new0  BranchType=C  Resistance=1.0  Inductance=1.0  SetiL0=off  InitialCurrent=0  Capacitance=Cs  Setx0=off  InitialVoltage=0  Measurements=None
  A : PMIOPort  Port=1  Side=Left
  B : PMIOPort  Port=2  Side=Left
  C : PMIOPort  Port=3  Side=Left
  "A " : PMIOPort  Port=4  Side=Right
  "B " : PMIOPort  Port=5  Side=Right
  "C " : PMIOPort  Port=6  Side=Right
  connections:
  A/RConn1 -- Ca/LConn1
  Ca/RConn1 -- "A "/RConn1
  B/RConn1 -- Cb/LConn1
  Cb/RConn1 -- "B "/RConn1
  C/RConn1 -- Cc/LConn1
  Cc/RConn1 -- "C "/RConn1

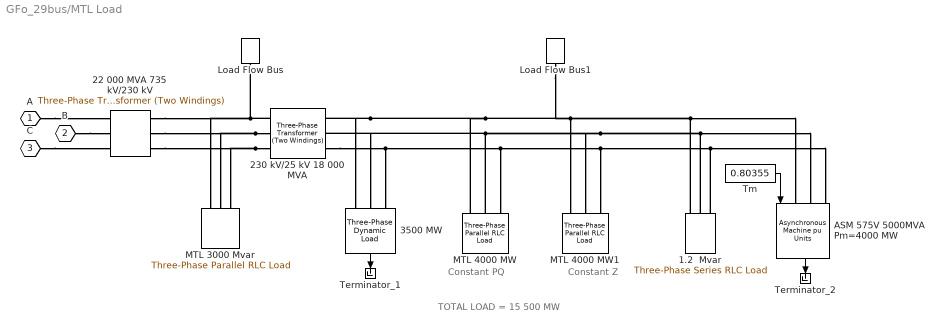
== system GFo_29bus/MTL Load ==
  note: Constant PQ
  note: Constant Z
  note: TOTAL LOAD = 15 500 MW
  1.2  Mvar : powerlib/Elements/Three-Phase Series RLC Load  LConnTagsString=A|B|C  Configuration=Y (grounded)  NominalVoltage=25e3  Vabc=[1e3 1e3 1e3]  Vabcp=[1e3 1e3 1e3]  NominalFrequency=60  UnbalancedPower=off  ActivePower=2000e6/50  InductivePower=0  CapacitivePower=2000e6  Pabc=[10e3 9e3 11e3]  QLabc=[100 90 110]  QCabc=[100 90 110]  Pabcp=[10e3 9e3 11e3]  QLabcp=[100 90 110]  QCabcp=[100 90 110]  Measurements=None  LoadType=constant Z
  22 000 MVA 735 kV/230 kV : powerlib/Elements/Three-Phase Transformer (Two Windings)  Winding1Connection=Yg  Winding2Connection=Delta (D1)  CoreType=Three single-phase transformers  SetSaturation=off  Hysteresis=off  DataFile='basic_model'  SetInitialFlux=off  Measurements=None  UNITS=pu  NominalPower=[ 22000e6 60 ]  Winding1="[ 735e3 0.002  0.12]"  Winding2=[230e3 0.002 0]  Rm=500  Lm=500  L0=0.5  Saturation="[ 0,0  ;  0.005,1.2  ;  1.0,1.4 ]"  InitialFluxes=[ 0.8 , -0.8 , 0.7 ]  MoreParameters=off  BreakLoop=off  DataType=off  TransfoNumber=0
  230 kV/25 kV 18 000 MVA : powerlib/Elements/Three-Phase Transformer (Two Windings)  Winding1Connection=Yg  Winding2Connection=Delta (D1)  CoreType=Three single-phase transformers  SetSaturation=off  Hysteresis=off  DataFile='basic_model'  SetInitialFlux=off  Measurements=None  UNITS=pu  NominalPower=[18000e6 60 ]  Winding1="[ 230e3  0.08/30   0.08 ]"  Winding2="[ 25e3  0.08/30  0.08]"  Rm=500  Lm=500  L0=0.5  Saturation="[ 0,0  ;  0.005,1.2  ;  1.0,1.4 ]"  InitialFluxes=[ 0.8 , -0.8 , 0.7 ]  MoreParameters=off  BreakLoop=off  DataType=off  TransfoNumber=0
  3500 MW : powerlib/Elements/Three-Phase Dynamic Load  NominalVoltage=[ 25e3 60 ]  ActiveReactivePowers=[3.5e+09 8.88178e-08]  PositiveSequence=[1.07643 -93.7608]  ExternalControl=off  NpNq="[1.5  2.5]"  TimeConstants="[0  0  0  0]"  MinimumVoltage=0.7  Tfilter=1e-4  LoadFlowParameters=[4,0,0,0,0]
      settings: SourceProductName=Simscape Power Systems  SourceProductBaseCode=PS
  ASM 575V 5000MVA Pm=4000 MW : powerlib/Machines/Asynchronous Machine pu Units  RotorType=Squirrel-cage  PresetModel=No  MechanicalLoad=Torque Tm  ShowDetailedParameters=on  ReferenceFrame=Rotor  Units=pu  MeasurementBus=off  NominalParameters="[5000e6 25e3  60]"  Stator=[0.01117 0.04832]  Rotor=[0.006 0.04832]  Cage1=[0.01909 0.0397]  Cage2=[0.01909 0.0397]  Lm=2.424  Mechanical="[1  0   2]"  PolePairs=2  InitialConditions=[0.00441886 0 0.895163 0.895163 0.895163 -126.28 -246.28 -6.27969]  SimulateSaturation=off  Saturation="[0.212,0.4201,0.8125,1.0979,1.4799,2.2457,3.2586,4.5763,6.4763 ;   0.5,0.7,0.9,1,1.1,1.2 ,1.3,1.4,1.5]"  LoadFlowParameters=0  TsPowergui=0  TsBlock=-1  IterativeModel=Trapezoidal non iterative  IterativeDiscreteModel=Trapezoidal non iterative  Pmec=4000000000
      settings: SourceProductName=Simscape Power Systems  SourceProductBaseCode=PS
  Load Flow Bus : powerlib/Measurements/Load Flow Bus  LConnTagsString=a  Phases=single  Connectors=on one side  ID=MTL2  Vbase=230e3  Vref=1  Vangle=0  VLF=1.092  VLFb=1  VLFc=1  angleLF=-56.7  angleLFb=0  angleLFc=0
      settings: AttributesFormatString=%<ID>\n%<Vbase>V\n%<VLF>pu\n%<angleLF>deg.  SourceProductName=Simscape Power Systems
  Load Flow Bus1 : powerlib/Measurements/Load Flow Bus  LConnTagsString=a  Phases=single  Connectors=on one side  ID=MTL_25  Vbase=25e3  Vref=1  Vangle=0  VLF=1.076  VLFb=1  VLFc=1  angleLF=-93.76  angleLFb=0  angleLFc=0
      settings: AttributesFormatString=%<ID>\n%<Vbase>V\n%<VLF>pu\n%<angleLF>deg.  SourceProductName=Simscape Power Systems
  MTL 3000 Mvar : powerlib/Elements/Three-Phase Parallel RLC Load  LConnTagsString=A|B|C  Configuration=Y (grounded)  NominalVoltage=230e3  Vabc=[1e3 1e3 1e3]  Vabcp=[1e3 1e3 1e3]  NominalFrequency=60  UnbalancedPower=off  ActivePower=0  InductivePower=0  CapacitivePower=3000e6  Pabc=[10e3 9e3 11e3]  QLabc=[100 90 110]  QCabc=[100 90 110]  Pabcp=[10e3 9e3 11e3]  QLabcp=[100 90 110]  QCabcp=[100 90 110]  Measurements=None  LoadType=constant Z
  MTL 4000 MW : powerlib/Elements/Three-Phase Parallel RLC Load  LConnTagsString=A|B|C  Configuration=Y (grounded)  NominalVoltage=(25000)*1.07643  Vabc=[1e3 1e3 1e3]  Vabcp=[1e3 1e3 1e3]  NominalFrequency=60  UnbalancedPower=off  ActivePower=4000000000  InductivePower=0  CapacitivePower=0  Pabc=[10e3 9e3 11e3]  QLabc=[100 90 110]  QCabc=[100 90 110]  Pabcp=[10e3 9e3 11e3]  QLabcp=[100 90 110]  QCabcp=[100 90 110]  Measurements=None  LoadType=constant PQ
  MTL 4000 MW1 : powerlib/Elements/Three-Phase Parallel RLC Load  LConnTagsString=A|B|C  Configuration=Y (grounded)  NominalVoltage=25e3  Vabc=[1e3 1e3 1e3]  Vabcp=[1e3 1e3 1e3]  NominalFrequency=60  UnbalancedPower=off  ActivePower=4000000000  InductivePower=0  CapacitivePower=0  Pabc=[10e3 9e3 11e3]  QLabc=[100 90 110]  QCabc=[100 90 110]  Pabcp=[10e3 9e3 11e3]  QLabcp=[100 90 110]  QCabcp=[100 90 110]  Measurements=None  LoadType=constant Z
  Terminator_1 : Terminator
  Terminator_2 : Terminator
  Tm : Constant  Value=0.80355
  A : PMIOPort  Port=1  Side=Left
  B : PMIOPort  Port=2  Side=Left
  C : PMIOPort  Port=3  Side=Left
  wires:
  Tm/1 -> ASM 575V 5000MVA Pm=4000 MW/1
  3500 MW/1 -> Terminator_1/1
  ASM 575V 5000MVA Pm=4000 MW/1 -> Terminator_2/1
  connections:
  A/RConn1 -- 22 000 MVA 735 kV/230 kV/LConn1
  B/RConn1 -- 22 000 MVA 735 kV/230 kV/LConn2
  C/RConn1 -- 22 000 MVA 735 kV/230 kV/LConn3
  230 kV/25 kV 18 000 MVA/LConn1 -- Load Flow Bus/LConn1 -- 22 000 MVA 735 kV/230 kV/RConn1 -- MTL 3000 Mvar/LConn1
  230 kV/25 kV 18 000 MVA/LConn2 -- 22 000 MVA 735 kV/230 kV/RConn2 -- MTL 3000 Mvar/LConn2
  230 kV/25 kV 18 000 MVA/LConn3 -- 22 000 MVA 735 kV/230 kV/RConn3 -- MTL 3000 Mvar/LConn3
  MTL 4000 MW1/LConn1 -- Load Flow Bus1/LConn1 -- MTL 4000 MW/LConn1 -- 230 kV/25 kV 18 000 MVA/RConn1 -- 3500 MW/LConn1 -- ASM 575V 5000MVA Pm=4000 MW/LConn1 -- 1.2  Mvar/LConn1
  MTL 4000 MW1/LConn2 -- MTL 4000 MW/LConn2 -- 230 kV/25 kV 18 000 MVA/RConn2 -- 3500 MW/LConn2 -- ASM 575V 5000MVA Pm=4000 MW/LConn2 -- 1.2  Mvar/LConn2
  230 kV/25 kV 18 000 MVA/RConn3 -- ASM 575V 5000MVA Pm=4000 MW/LConn3 -- 1.2  Mvar/LConn3 -- MTL 4000 MW1/LConn3 -- MTL 4000 MW/LConn3 -- 3500 MW/LConn3

== system GFo_29bus/Model Initialization ==
